simulink model "exp2"  (R2025b)
settings: Solver=VariableStepAuto  StartTime=0.0  StopTime=10.0  RelTol=1e-3
settings Model: Creator=SUBHASH  LastModifiedBy=SUBHASH

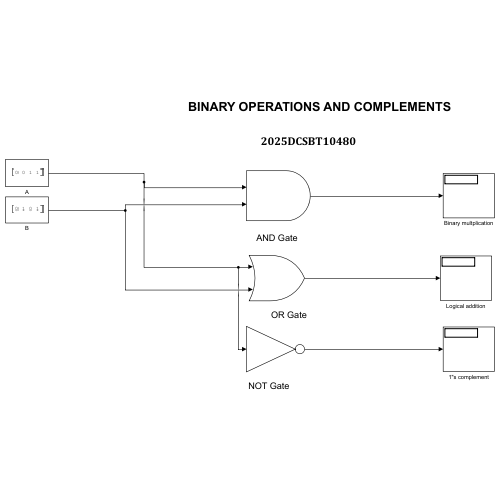
[thumbnail: Simulink's stored preview of the top-level diagram]
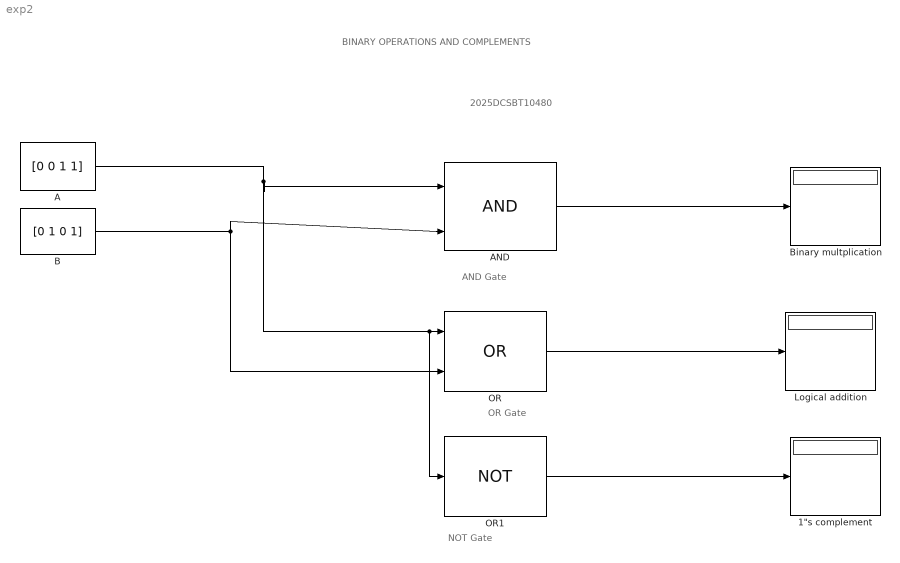
== system exp2 ==
  note: NOT Gate
  note: OR Gate
  note: AND Gate
  note: BINARY OPERATIONS AND COMPLEMENTS
  note: 2025DCSBT10480
  "1\"s complement" : Display
  A : Constant  Value=[0 0 1 1]
  AND : Logic  IconShape=distinctive  AllPortsSameDT=off  OutDataTypeStr=boolean
  B : Constant  Value=[0 1 0 1]
  Binary multplication : Display
  Logical addition : Display
  OR : Logic  Operator=OR  IconShape=distinctive  AllPortsSameDT=off  OutDataTypeStr=boolean
  OR1 : Logic  Operator=NOT  IconShape=distinctive  AllPortsSameDT=off  OutDataTypeStr=boolean
  wires:
  A/1 -> OR1/1, OR/1, AND/1
  B/1 -> OR/2, AND/2
  AND/1 -> Binary multplication/1
  OR/1 -> Logical addition/1
  OR1/1 -> "1\"s complement"/1
